simulink model "quadcopter_breach"  (R2018b)
settings: Solver=FixedStepAuto  StartTime=0.0  StopTime=tspan(end)  FixedStep=options.dt  RelTol=1e-3
undefined symbols (not defined in the file): options
libraries: neural x136, simulink x3
(part 6 of 6)

== system quadcopter_breach/NN_cex_1/Layer 3/Delays 1 ==
  "p{3}" : Inport  PortDimensions=30
      mask Display: e = 0.06;c1 = [120 230 180]/255;c2 = ([120 230 180]+0)/(256+128);c3 = ([120 230 180]+128)/(256+128);patch([0 1 1 0],[0 0 1 1],c1);patch([0 1 1 1-e 1-e 0+e],[0 0 1 1-e 0+e 0+e],c2);patch([0 0 1 1-e 0+e 0+e],[0 1 1 1-e 1-e 0+e],c3);plot([0 1 1 0 0],[0 0 1 1 0]);
  mux : Mux  Inputs=1
      mask Display: e = 0.06;c1 = [120 150 230]/255;c2 = ([120 150 230]+0)/383;c3 = ([120 150 230]+128)/383;patch([0 1 1 0],[0 0 1 1],c1);patch([0 1 1 1-e 1-e 0+e],[0 0 1 1-e 0+e 0+e],c2);patch([0 0 1 1-e 0+e 0+e],[0 1 1 1-e 1-e 0+e],c3);plot([0 1 1 0 0],[0 0 1 1 0]);disp('Mux')
  "pd{3,2}" : Outport
      mask Display: e = 0.06;c1 = [120 230 180]/255;c2 = ([120 230 180]+0)/(256+128);c3 = ([120 230 180]+128)/(256+128);patch([0 1 1 0],[0 0 1 1],c1);patch([0 1 1 1-e 1-e 0+e],[0 0 1 1-e 0+e 0+e],c2);patch([0 0 1 1-e 0+e 0+e],[0 1 1 1-e 1-e 0+e],c3);plot([0 1 1 0 0],[0 0 1 1 0]);
  wires:
  "p{3}"/1 -> mux/1
  mux/1 -> "pd{3,2}"/1

== system quadcopter_breach/NN_cex_1/Layer 3/LW{3,2} ==
  "ad{3,2}" : Inport  PortDimensions=30
      mask Display: e = 0.06;c1 = [120 230 180]/255;c2 = ([120 230 180]+0)/(256+128);c3 = ([120 230 180]+128)/(256+128);patch([0 1 1 0],[0 0 1 1],c1);patch([0 1 1 1-e 1-e 0+e],[0 0 1 1-e 0+e 0+e],c2);patch([0 0 1 1-e 0+e 0+e],[0 1 1 1-e 1-e 0+e],c3);plot([0 1 1 0 0],[0 0 1 1 0]);
  "IW{3,2}(1,:)'" : Constant  Value=[0.373172652347722400012486332343542017042636871337890625;0.043679932730451252742565060316337621770799160003662109375;0.07664903965921961159768471816278179176151752471923828125;-0.040612701834875704343108537841544602997601032257080078125;-0.30143636959132147357109943186515010893344879150390625;-0.48101400860255727476300080525106750428676605224609375;-0.035178314776622525428262377999999444000422954559326171875;0.06961339828498173953885697073928895406424999237060546875;-0.07941176068149512212723806214853539131581783294677734375;-0.022026622465605293077484105879193521104753017425537109375;0.0233844162198706718991392250472927116788923740386962890625;0.39667605204551026343295916376519016921520233154296875;0.04670989481239018470404289473663084208965301513671875;0.0312105237739146723630057067566667683422565460205078125;-0.36667833681907902043661806601448915898799896240234375;-0.003500935526659935438653636907702093594707548618316650390625;-0.16489828784776705550285669232835061848163604736328125;-0.0883268539312018763354217298910953104496002197265625;0.02533843341297815909829438396627665497362613677978515625;-0.0512078225569689016172247875147149898111820220947265625;-0.031884881480663547492770959479457815177738666534423828125;0.772210618834126005793905278551392257213592529296875;0.4393289290664912360995231210836209356784820556640625;-0.08571305859992249531753572000525309704244136810302734375;-0.0713761216850390400878723085043020546436309814453125;-0.13420108410834663548172329683438874781131744384765625;0.00963425063069851643493546333729682373814284801483154296875;-0.8344739818400135344944601456518284976482391357421875;0.07354779756570963000772422901718528009951114654541015625;-0.03085167611031014445188702666200697422027587890625]
      mask Display: e = 0.06;c1 = [120 150 230]/255;c2 = ([120 150 230]+0)/383;c3 = ([120 150 230]+128)/383;patch([0 1 1 0],[0 0 1 1],c1);patch([0 1 1 1-e 1-e 0+e],[0 0 1 1-e 0+e 0+e],c2);patch([0 0 1 1-e 0+e 0+e],[0 1 1 1-e 1-e 0+e],c3);plot([0 1 1 0 0],[0 0 1 1 0]);disp('weights');
  Mux : Mux  Inputs=1
      mask Display: e = 0.06;c1 = [120 150 230]/255;c2 = ([120 150 230]+0)/383;c3 = ([120 150 230]+128)/383;patch([0 1 1 0],[0 0 1 1],c1);patch([0 1 1 1-e 1-e 0+e],[0 0 1 1-e 0+e 0+e],c2);patch([0 0 1 1-e 0+e 0+e],[0 1 1 1-e 1-e 0+e],c3);plot([0 1 1 0 0],[0 0 1 1 0]);disp('Mux');
  dotprod1 : neural/Weight Functions/dotprod
  "lz{3,2}" : Outport
      mask Display: e = 0.06;c1 = [120 230 180]/255;c2 = ([120 230 180]+0)/(256+128);c3 = ([120 230 180]+128)/(256+128);patch([0 1 1 0],[0 0 1 1],c1);patch([0 1 1 1-e 1-e 0+e],[0 0 1 1-e 0+e 0+e],c2);patch([0 0 1 1-e 0+e 0+e],[0 1 1 1-e 1-e 0+e],c3);plot([0 1 1 0 0],[0 0 1 1 0]);
  wires:
  "IW{3,2}(1,:)'"/1 -> dotprod1/1
  "ad{3,2}"/1 -> dotprod1/2
  dotprod1/1 -> Mux/1
  Mux/1 -> "lz{3,2}"/1

== matlab function quadcopter_breach/MATLAB Function ==
  data: r1 input; F output; r2 input; r3 input; x3 input; x6 input; x7 input; x8 input; x10 input; x11 input; tau_phi output; tau_theta output; tau_psi output
function [F,tau_phi,tau_theta,tau_psi] = fcn(r1,r2,r3,x3,x6,x7,x8,x10,x11)
%initialization
m=1.4;
g=9.81;
F= m*g-10*(x3-r1)+3*x6;
tau_phi=-(x7-r2)-x10;
tau_theta=-(x8-r3)-x11;
tau_psi=0;
